simulink model "DCDC5to14"  (R2022a)
settings: Solver=VariableStepAuto  StartTime=0.0  StopTime=0.01  RelTol=1e-3
libraries: spsCurrentMeasurementLib x4, spsSeriesRLCBranchLib x3, spsVoltageMeasurementLib x2, spsDCVoltageSourceLib x1, spsDiodeLib x1, spsMosfetLib x1, spsPWMGeneratorDCDCLib x1, dspmathops x1, spsSawtoothGeneratorLib x1, msbUtilities x1, spspowerguiLib x1
settings Model: Creator=jack  LastModifiedBy=jack

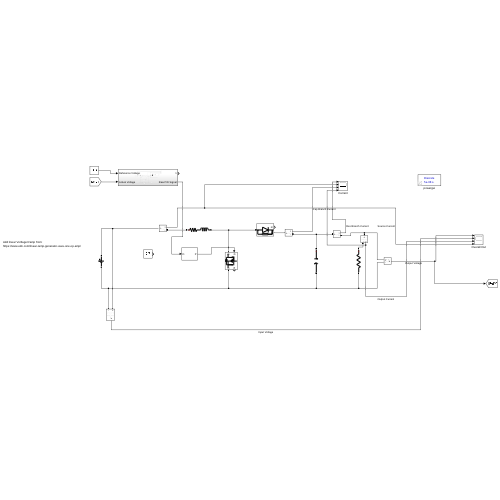
[thumbnail: Simulink's stored preview of the top-level diagram]
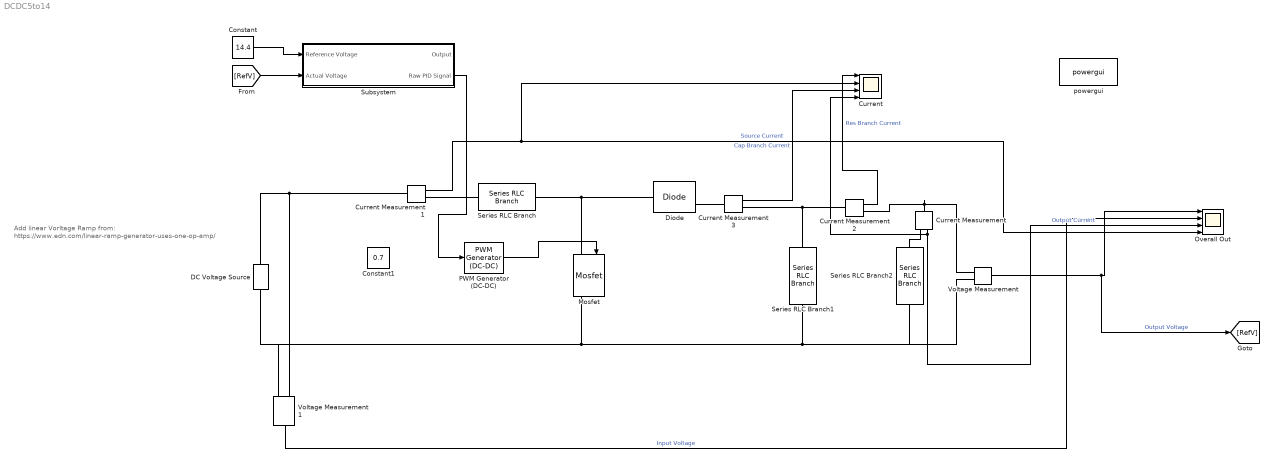
== system DCDC5to14 ==
  note: Add linear Vorltage Ramp from:
      | https://www.edn.com/linear-ramp-generator-uses-one-op-amp/
  Constant : Constant  Value=14.4
  Constant1 : Constant  Value=0.7
  Current : Scope  NumInputPorts=4
  Current Measurement{,1..3} (4 alike) : spsCurrentMeasurementLib/Current Measurement  PhasorSimulation=off  OutputType=Complex  PSBequivalent=0
  DC Voltage Source : spsDCVoltageSourceLib/DC Voltage Source  Amplitude=5  Measurements=None
  Diode : spsDiodeLib/Diode  Ron=0.001  Lon=0  Vf=0.42  IC=0  UseSnubber=0  Rs=500  Cs=250e-9  Measurements=on
  Mosfet : spsMosfetLib/Mosfet  Ron=0.1  Lon=0  Rd=0.01  Vfd=0.5  IC=0  Rs=1e5  Cs=inf  Measurements=on
  Overall Out : Scope  NumInputPorts=4
  PWM Generator (DC-DC) : spsPWMGeneratorDCDCLib/PWM Generator (DC-DC)  Fsw=100e3  Ts=0
  Series RLC Branch : spsSeriesRLCBranchLib/Series RLC Branch  LConnTagsString=__new0  RConnTagsString=__new0  BranchType=RL  Resistance=0  Inductance=28.33e-6  SetiL0=off  InitialCurrent=0  Capacitance=1e-9  Setx0=off  InitialVoltage=0  Measurements=None
  Series RLC Branch1 : spsSeriesRLCBranchLib/Series RLC Branch  LConnTagsString=__new0  RConnTagsString=__new0  BranchType=C  Resistance=1  Inductance=1e-3  SetiL0=off  InitialCurrent=0  Capacitance=10e-6  Setx0=off  InitialVoltage=0  Measurements=None
  Series RLC Branch2 : spsSeriesRLCBranchLib/Series RLC Branch  LConnTagsString=__new0  RConnTagsString=__new0  BranchType=R  Resistance=12  Inductance=1e-3  SetiL0=off  InitialCurrent=0  Capacitance=1e-6  Setx0=off  InitialVoltage=0  Measurements=None
  Subsystem : Subsystem
  Voltage Measurement : spsVoltageMeasurementLib/Voltage Measurement  PhasorSimulation=off  OutputType=Complex  PSBequivalent=0
  Voltage Measurement1 : spsVoltageMeasurementLib/Voltage Measurement  PhasorSimulation=off  OutputType=Complex  PSBequivalent=0
  powergui : spspowerguiLib/powergui  Priority=1  SimulationMode=Discrete  SampleTime=50e-9  frequency=60  Iterations=50  frequencyindice=0  Pbase=100e6  ErrMax=1e-4  UnitsV=kV  UnitsW=MW  buscounter=0  FunctionMessages=off  echomessages=off  EnableUseOfTLC=off  CurrentSourceSwitches=off  DisableSnubberDevices=off  DisableRonSwitches=off  DisableVfSwitches=off  DisplayEquations=off  AutomaticDiscreteSolvers=off  SolverType=Tustin/Backward Euler (TBE)  Interpol=off  ExternalGateDelay=off  methode=off  Ts=100  x0status=blocks  SPID=on  SwTol=0  HookPort=off  NonlinearTolerance=1e-4  nMaxIteration=100  ContinueOnMaxIteration=off  RestoreLinks=warning  ResistiveCurrentMeasurement=off  Frange=[0:2:500]  Ylog=off  Xlog=on  ShowGrid=off  save=off  variable=ZData  structure=0  ZoomFFT=off  StartTime=0.0  cycles=1  DisplayStyle=1  fundamental=60  FreqAxis=off  MaxFrequency=1000  frequencyindicesteady=1  RmsSteady=1  display=off
  wires:
  Voltage Measurement/1 -> [RefV], Overall Out/1  "Output Voltage"
  Voltage Measurement1/1 -> Overall Out/2  "Input Voltage"
  Current Measurement/1 -> Overall Out/3, Current/4  "Output Current"
  Current Measurement1/1 -> Current/2, Overall Out/4  "Source Current"
  Current Measurement2/1 -> Current/1  "Res Branch Current"
  Current Measurement3/1 -> Current/3  "Cap Branch Current"
  [RefV] -> Subsystem/2(Actual Voltage)
  Constant/1 -> Subsystem/1(Reference Voltage)
  Subsystem/2(Raw PID Signal) -> PWM Generator (DC-DC)/1
  PWM Generator (DC-DC)/1 -> Mosfet/1
  connections:
  Diode/LConn1 -- Mosfet/LConn1 -- Series RLC Branch/RConn1
  Current Measurement/LConn1 -- Voltage Measurement/LConn1 -- Current Measurement2/RConn1
  Series RLC Branch1/RConn1 -- Voltage Measurement/LConn2 -- Series RLC Branch2/RConn1 -- Voltage Measurement1/LConn2 -- DC Voltage Source/LConn1 -- Mosfet/RConn1
  Current Measurement/RConn1 -- Series RLC Branch2/LConn1
  Current Measurement1/RConn1 -- Series RLC Branch/LConn1
  DC Voltage Source/RConn1 -- Current Measurement1/LConn1 -- Voltage Measurement1/LConn1
  Current Measurement2/LConn1 -- Current Measurement3/RConn1 -- Series RLC Branch1/LConn1
  Diode/RConn1 -- Current Measurement3/LConn1

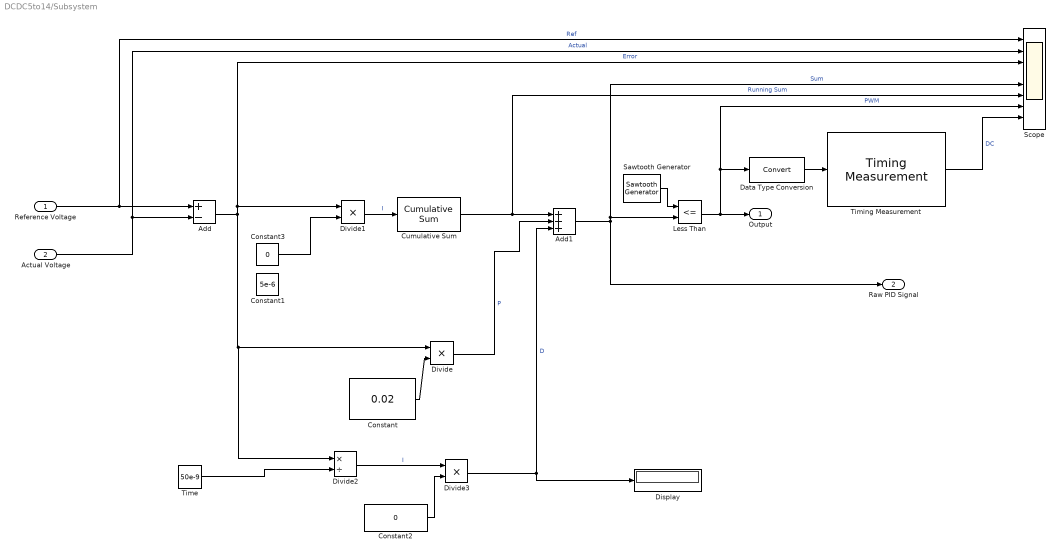
== system DCDC5to14/Subsystem ==
  Reference Voltage : Inport
  Actual Voltage : Inport  Port=2
  Add : Sum  Inputs=+-
  Add1 : Sum  Inputs=+++
  Constant : Constant  Value=0.02
  Constant1 : Constant  Value=5e-6  SampleTime=50e-6
  Constant2 : Constant  Value=0
  Constant3 : Constant  Value=0
  Cumulative Sum : dspmathops/Cumulative Sum  dim=Channels (running sum)  InputProcessing=Columns as channels (frame based)  reset_popup=None  roundingMode=Floor  overflowMode=off  outputDataTypeStr=Inherit: Same as accumulator  outputMin=[]  outputMax=[]  outputLastDataTypeStr=Inherit: Same as accumulator
  Data Type Conversion : DataTypeConversion  SaturateOnIntegerOverflow=off  RndMeth=Floor
  Display : Display
  Divide : Product  Inputs=**
  Divide1 : Product  Inputs=**
  Divide2 : Product  Inputs=*/
  Divide3 : Product  Inputs=**
  Less Than : RelationalOperator  Operator=<=  OutDataTypeStr=boolean  RndMeth=Simplest  InputSameDT=off
  Sawtooth Generator : spsSawtoothGeneratorLib/Sawtooth Generator  Freq=50e3  Phase=180  Ts=0
  Scope : Scope  NumInputPorts=8
  Time : Constant  Value=50e-9
  Timing Measurement : msbUtilities/Timing Measurement  Period=off  Frequency=off  RiseTime=off  FallTime=off  DutyCycle=on  Delay=off  SameRefThreshold=on  GlobalRefThreshold=0  Range=[-1 1]  MeasurementType=80% / 20%  ThresholdMax=0.6  ThresholdMin=-0.6  DcRefThreshold=0  DelayRefThreshold=0  DelayTstThreshold=0
      settings: SourceProductBaseCode=AM
  Output : Outport
  Raw PID Signal : Outport  Port=2
  wires:
  Reference Voltage/1 -> Scope/1, Add/1  "Ref"
  Actual Voltage/1 -> Scope/2, Add/2  "Actual"
  Add/1 -> Divide2/1, Divide/1, Divide1/1, Scope/3  "Error"
  Constant/1 -> Divide/2
  Sawtooth Generator/1 -> Less Than/1
  Add1/1 -> Raw PID Signal/1, Scope/5, Less Than/2  "Sum"
  Less Than/1 -> Data Type Conversion/1, Scope/7, Output/1  "PWM"
  Timing Measurement/1 -> Scope/8  "DC"
  Data Type Conversion/1 -> Timing Measurement/1
  Divide1/1 -> Cumulative Sum/1  "I"
  Cumulative Sum/1 -> Add1/1, Scope/6  "Running Sum"
  Divide/1 -> Add1/2  "P"
  Time/1 -> Divide2/2
  Divide3/1 -> Display/1, Add1/3  "D"
  Divide2/1 -> Divide3/1  "I"
  Constant2/1 -> Divide3/2
  Constant3/1 -> Divide1/2
